simulink model "currency2"  (R2023b)
settings: Solver=VariableStepAuto  StartTime=0.0  StopTime=10.0  RelTol=1e-3
libraries: visionsources x1
settings Model: Creator=ROHIT  LastModifiedBy=ROHIT
settings SFSimCC: SimTargetLang=C++

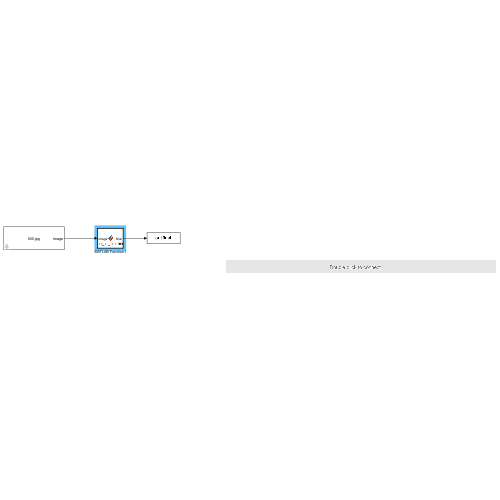
[thumbnail: Simulink's stored preview of the top-level diagram]
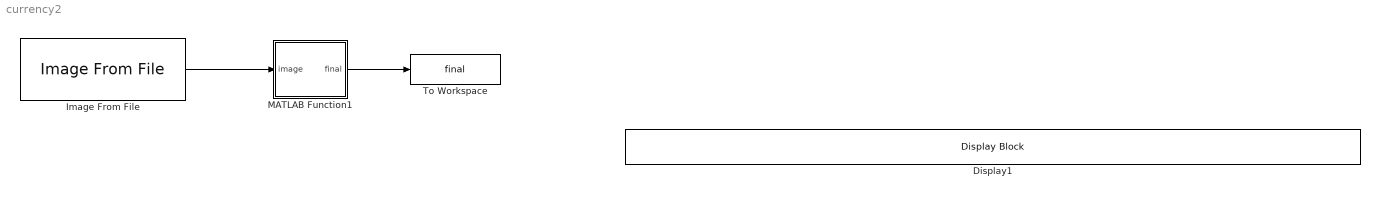
== system currency2 ==
  Display1 : DisplayBlock  LabelPosition=Hide  Transparency=1
  Image From File : visionsources/Image From File  Tag=vipblks_nd  FileName=G:\Downloads\500.jpg  Ts=inf  imagePorts=One multidimensional signal  OutPortLabels=R|G|B  ImageDataType=Inherit from input image  sdImageDataType=uint(8)  Signed=on  WordLength=16  FractionLengthMode=User-defined  FractionLength=15
  MATLAB Function1 : MATLAB Function  TreatAsAtomicUnit=on
  To Workspace : ToWorkspace  VariableName=final  SampleTime=-1
  wires:
  MATLAB Function1/1(final) -> To Workspace/1
  Image From File/1 -> MATLAB Function1/1(image)

== matlab function currency2/MATLAB Function1 ==
  data: final output; image input
function final = ocr_in_simulink(image)
    gray_image = im2gray(image);

    % Resize the grayscale image 
    resized_image = imresize(gray_image, 0.5);
    binary_image = imbinarize(resized_image);

    % Perform OCR on the binary image
    txt1 = ocr(binary_image, 'CharacterSet', '0125', 'TextLayout', 'Block');

    % Extract the text from the OCR results
    extracted_text = {txt1.Text}; % Convert to cell array

    % Concatenate all extracted text
    final1 = strjoin(extracted_text, '');
    final1 = string(final1);
    
    
    disp(final1);
    final = str2double(final1);
end
